simulink model "IK_PickPlaceTrajectory"  (R2023a)
settings: Solver=VariableStepAuto  StartTime=0.0  StopTime=10.0  RelTol=1e-3
values from neighbouring files (symbols this model uses):
  m = [4.043687892216430,4.088351020081470,2.975514330882000,2.005251413706830,1.580964077451070,0.312204788418883]    [Alternative_Approach_for_Jacobian.m]    (also in Dynamics6DOF_code.m)
undefined symbols (not defined in the file or in its folder): B, Spline, X, Y, Z
libraries: sm_lib x61, nesl_utility x19, robotcorelib x3, robotmaniplib x1
(part 2 of 2)

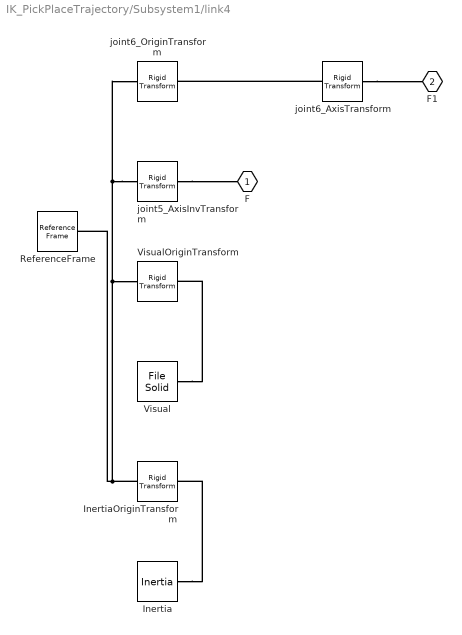
== system IK_PickPlaceTrajectory/Subsystem1/link4 ==
  Inertia : sm_lib/Body Elements/Inertia  InertiaType=Custom  Mass=1.93952788406336  MassUnits=kg  CenterOfMass=[0, 0, 0]  CenterOfMassUnits=m  MomentsOfInertia=[0.00155390886602976, 0.00197625240925502, 0.00139914012504898]  MomentsOfInertiaUnits=kg*m^2  ProductsOfInertia=[-0.000238629251977827, 2.66730188215764e-06, -2.69206560401887e-06]  ProductsOfInertiaUnits=kg*m^2  GraphicType=None  MarkerShape=Inertia  MarkerSize=20  GraphicVisPropType=SimpleVisualProperties  GraphicDiffuseColor=[0.5 0.5 0.5]  GraphicSpecularColor=[0.5 0.5 0.5 1.0]  GraphicAmbientColor=[0.15 0.15 0.15 1.0]  GraphicEmissiveColor=[0.0 0.0 0.0 1.0]  GraphicShininess=75  GraphicOpacity=1.0
  InertiaOriginTransform : sm_lib/Frames and Transforms/Rigid Transform  TranslationMethod=Cartesian  TranslationStandardOffset=0  TranslationStandardOffsetUnits=m  TranslationStandardAxis=+Z  TranslationCartesianOffset=[0.00193589454404341, 0.0412277276852661, -0.00711984165498196]  TranslationCartesianOffsetUnits=m  TranslationROffset=0  TranslationROffsetUnits=m  TranslationZOffset=0  TranslationZOffsetUnits=m  TranslationThetaOffset=0  TranslationThetaOffsetUnits=deg  RotationMethod=RotationSequence  RotationAngleUnits=deg  RotationStandardAxis=+Z  RotationAngle=0.0  RotationArbitraryAxis=[0 0 1]  FollAlignAxisA=+X  BaseAlignAxisA=+Y  FollAlignAxisB=+Y  BaseAlignAxisB=+Z  RotationSequenceAxes=BaseAxes  RotationSequence=XYZ  RotationSequenceAngles=[0, 0, 0]  RotationSequenceAnglesUnits=rad  RotationMatrix=[1 0 0; 0 1 0; 0 0 1]  Quaternion=[1 0 0 0]
  ReferenceFrame : sm_lib/Frames and Transforms/Reference Frame
  Visual : sm_lib/Body Elements/File Solid  ExtGeomFileName=PickandPlace_Assembly/meshes/link4.STL  UnitType=Custom  ExtGeomFileUnits=m  StepReaderType=HEX  ExportConvexHullGeometry=off  InertiaType=Custom  Mass=0  MassUnits=kg  CenterOfMass=[0, 0, 0]  CenterOfMassUnits=m  MomentsOfInertia=[0, 0, 0]  MomentsOfInertiaUnits=kg*m^2  ProductsOfInertia=[0, 0, 0]  ProductsOfInertiaUnits=kg*m^2  BasedOnType=DensityFromFile  Density=1000  DensityUnits=kg/m^3  DoExposeReferenceFrame=on  SerializedFrames=<Frames/>  GraphicType=FromGeometry  MarkerShape=Sphere  MarkerSize=10  GraphicVisPropType=SimpleVisualProperties  GraphicDiffuseColor=[0.752941176470588, 0.752941176470588, 0.752941176470588]  GraphicSpecularColor=[0.5 0.5 0.5 1.0]  GraphicAmbientColor=[0.15 0.15 0.15 1.0]  GraphicEmissiveColor=[0.0 0.0 0.0 1.0]  GraphicShininess=75  GraphicOpacity=1
  VisualOriginTransform : sm_lib/Frames and Transforms/Rigid Transform  TranslationMethod=Cartesian  TranslationStandardOffset=0  TranslationStandardOffsetUnits=m  TranslationStandardAxis=+Z  TranslationCartesianOffset=[0, 0, 0.132]  TranslationCartesianOffsetUnits=m  TranslationROffset=0  TranslationROffsetUnits=m  TranslationZOffset=0  TranslationZOffsetUnits=m  TranslationThetaOffset=0  TranslationThetaOffsetUnits=deg  RotationMethod=RotationSequence  RotationAngleUnits=deg  RotationStandardAxis=+Z  RotationAngle=0.0  RotationArbitraryAxis=[0 0 1]  FollAlignAxisA=+X  BaseAlignAxisA=+Y  FollAlignAxisB=+Y  BaseAlignAxisB=+Z  RotationSequenceAxes=BaseAxes  RotationSequence=XYZ  RotationSequenceAngles=[0, 0, 0]  RotationSequenceAnglesUnits=rad  RotationMatrix=[1 0 0; 0 1 0; 0 0 1]  Quaternion=[1 0 0 0]
  joint5_AxisInvTransform : sm_lib/Frames and Transforms/Rigid Transform  TranslationMethod=Cartesian  TranslationStandardOffset=0  TranslationStandardOffsetUnits=m  TranslationStandardAxis=+Z  TranslationCartesianOffset=[0, 0, 0]  TranslationCartesianOffsetUnits=m  TranslationROffset=0  TranslationROffsetUnits=m  TranslationZOffset=0  TranslationZOffsetUnits=m  TranslationThetaOffset=0  TranslationThetaOffsetUnits=deg  RotationMethod=ArbitraryAxis  RotationAngleUnits=rad  RotationStandardAxis=+Z  RotationAngle=0  RotationArbitraryAxis=[1, 0, 0]  FollAlignAxisA=+X  BaseAlignAxisA=+Y  FollAlignAxisB=+Y  BaseAlignAxisB=+Z  RotationSequenceAxes=FollowerAxes  RotationSequence=XYX  RotationSequenceAngles=[0 0 0]  RotationSequenceAnglesUnits=deg  RotationMatrix=[1 0 0; 0 1 0; 0 0 1]  Quaternion=[1 0 0 0]
  joint6_AxisTransform : sm_lib/Frames and Transforms/Rigid Transform  TranslationMethod=Cartesian  TranslationStandardOffset=0  TranslationStandardOffsetUnits=m  TranslationStandardAxis=+Z  TranslationCartesianOffset=[0, 0, 0]  TranslationCartesianOffsetUnits=m  TranslationROffset=0  TranslationROffsetUnits=m  TranslationZOffset=0  TranslationZOffsetUnits=m  TranslationThetaOffset=0  TranslationThetaOffsetUnits=deg  RotationMethod=ArbitraryAxis  RotationAngleUnits=rad  RotationStandardAxis=+Z  RotationAngle=0  RotationArbitraryAxis=[1, 0, 0]  FollAlignAxisA=+X  BaseAlignAxisA=+Y  FollAlignAxisB=+Y  BaseAlignAxisB=+Z  RotationSequenceAxes=FollowerAxes  RotationSequence=XYX  RotationSequenceAngles=[0 0 0]  RotationSequenceAnglesUnits=deg  RotationMatrix=[1 0 0; 0 1 0; 0 0 1]  Quaternion=[1 0 0 0]
  joint6_OriginTransform : sm_lib/Frames and Transforms/Rigid Transform  TranslationMethod=Cartesian  TranslationStandardOffset=0  TranslationStandardOffsetUnits=m  TranslationStandardAxis=+Z  TranslationCartesianOffset=[0, 0, 0.132]  TranslationCartesianOffsetUnits=m  TranslationROffset=0  TranslationROffsetUnits=m  TranslationZOffset=0  TranslationZOffsetUnits=m  TranslationThetaOffset=0  TranslationThetaOffsetUnits=deg  RotationMethod=RotationSequence  RotationAngleUnits=deg  RotationStandardAxis=+Z  RotationAngle=0.0  RotationArbitraryAxis=[0 0 1]  FollAlignAxisA=+X  BaseAlignAxisA=+Y  FollAlignAxisB=+Y  BaseAlignAxisB=+Z  RotationSequenceAxes=BaseAxes  RotationSequence=XYZ  RotationSequenceAngles=[-1.5707963267949, 0, 0]  RotationSequenceAnglesUnits=rad  RotationMatrix=[1 0 0; 0 1 0; 0 0 1]  Quaternion=[1 0 0 0]
  F : PMIOPort  Side=Left
  F1 : PMIOPort  Port=2  Side=Right
  connections:
  Inertia/RConn1 -- InertiaOriginTransform/RConn1
  joint5_AxisInvTransform/LConn1 -- joint6_OriginTransform/LConn1 -- InertiaOriginTransform/LConn1 -- ReferenceFrame/RConn1 -- VisualOriginTransform/LConn1
  Visual/RConn1 -- VisualOriginTransform/RConn1
  joint5_AxisInvTransform/RConn1 -- F/RConn1
  joint6_AxisTransform/RConn1 -- F1/RConn1
  joint6_AxisTransform/LConn1 -- joint6_OriginTransform/RConn1

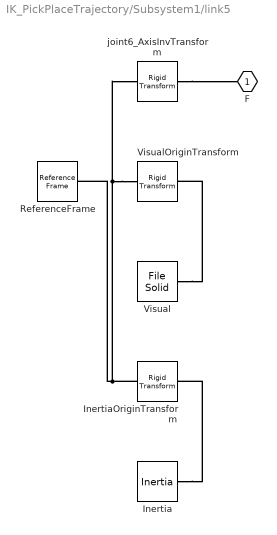
== system IK_PickPlaceTrajectory/Subsystem1/link5 ==
  Inertia : sm_lib/Body Elements/Inertia  InertiaType=Custom  Mass=0.312204788121022  MassUnits=kg  CenterOfMass=[0, 0, 0]  CenterOfMassUnits=m  MomentsOfInertia=[0.000111486628802788, 0.00017220756532504, 0.000149930296123144]  MomentsOfInertiaUnits=kg*m^2  ProductsOfInertia=[-2.62510399493773e-06, -6.16294543592803e-07, 1.09193037299933e-05]  ProductsOfInertiaUnits=kg*m^2  GraphicType=None  MarkerShape=Inertia  MarkerSize=20  GraphicVisPropType=SimpleVisualProperties  GraphicDiffuseColor=[0.5 0.5 0.5]  GraphicSpecularColor=[0.5 0.5 0.5 1.0]  GraphicAmbientColor=[0.15 0.15 0.15 1.0]  GraphicEmissiveColor=[0.0 0.0 0.0 1.0]  GraphicShininess=75  GraphicOpacity=1.0
  InertiaOriginTransform : sm_lib/Frames and Transforms/Rigid Transform  TranslationMethod=Cartesian  TranslationStandardOffset=0  TranslationStandardOffsetUnits=m  TranslationStandardAxis=+Z  TranslationCartesianOffset=[0.000634869948304639, 0.00391637711045545, 0.0604907685184927]  TranslationCartesianOffsetUnits=m  TranslationROffset=0  TranslationROffsetUnits=m  TranslationZOffset=0  TranslationZOffsetUnits=m  TranslationThetaOffset=0  TranslationThetaOffsetUnits=deg  RotationMethod=RotationSequence  RotationAngleUnits=deg  RotationStandardAxis=+Z  RotationAngle=0.0  RotationArbitraryAxis=[0 0 1]  FollAlignAxisA=+X  BaseAlignAxisA=+Y  FollAlignAxisB=+Y  BaseAlignAxisB=+Z  RotationSequenceAxes=BaseAxes  RotationSequence=XYZ  RotationSequenceAngles=[0, 0, 0]  RotationSequenceAnglesUnits=rad  RotationMatrix=[1 0 0; 0 1 0; 0 0 1]  Quaternion=[1 0 0 0]
  ReferenceFrame : sm_lib/Frames and Transforms/Reference Frame
  Visual : sm_lib/Body Elements/File Solid  ExtGeomFileName=PickandPlace_Assembly/meshes/link5.STL  UnitType=Custom  ExtGeomFileUnits=m  StepReaderType=HEX  ExportConvexHullGeometry=off  InertiaType=Custom  Mass=0  MassUnits=kg  CenterOfMass=[0, 0, 0]  CenterOfMassUnits=m  MomentsOfInertia=[0, 0, 0]  MomentsOfInertiaUnits=kg*m^2  ProductsOfInertia=[0, 0, 0]  ProductsOfInertiaUnits=kg*m^2  BasedOnType=DensityFromFile  Density=1000  DensityUnits=kg/m^3  DoExposeReferenceFrame=on  SerializedFrames=<Frames/>  GraphicType=FromGeometry  MarkerShape=Sphere  MarkerSize=10  GraphicVisPropType=SimpleVisualProperties  GraphicDiffuseColor=[0.752941176470588, 0.752941176470588, 0.752941176470588]  GraphicSpecularColor=[0.5 0.5 0.5 1.0]  GraphicAmbientColor=[0.15 0.15 0.15 1.0]  GraphicEmissiveColor=[0.0 0.0 0.0 1.0]  GraphicShininess=75  GraphicOpacity=1
  VisualOriginTransform : sm_lib/Frames and Transforms/Rigid Transform  TranslationMethod=Cartesian  TranslationStandardOffset=0  TranslationStandardOffsetUnits=m  TranslationStandardAxis=+Z  TranslationCartesianOffset=[0, 0, 0.050999]  TranslationCartesianOffsetUnits=m  TranslationROffset=0  TranslationROffsetUnits=m  TranslationZOffset=0  TranslationZOffsetUnits=m  TranslationThetaOffset=0  TranslationThetaOffsetUnits=deg  RotationMethod=RotationSequence  RotationAngleUnits=deg  RotationStandardAxis=+Z  RotationAngle=0.0  RotationArbitraryAxis=[0 0 1]  FollAlignAxisA=+X  BaseAlignAxisA=+Y  FollAlignAxisB=+Y  BaseAlignAxisB=+Z  RotationSequenceAxes=BaseAxes  RotationSequence=XYZ  RotationSequenceAngles=[0, 0, 0]  RotationSequenceAnglesUnits=rad  RotationMatrix=[1 0 0; 0 1 0; 0 0 1]  Quaternion=[1 0 0 0]
  joint6_AxisInvTransform : sm_lib/Frames and Transforms/Rigid Transform  TranslationMethod=Cartesian  TranslationStandardOffset=0  TranslationStandardOffsetUnits=m  TranslationStandardAxis=+Z  TranslationCartesianOffset=[0, 0, 0]  TranslationCartesianOffsetUnits=m  TranslationROffset=0  TranslationROffsetUnits=m  TranslationZOffset=0  TranslationZOffsetUnits=m  TranslationThetaOffset=0  TranslationThetaOffsetUnits=deg  RotationMethod=ArbitraryAxis  RotationAngleUnits=rad  RotationStandardAxis=+Z  RotationAngle=0  RotationArbitraryAxis=[1, 0, 0]  FollAlignAxisA=+X  BaseAlignAxisA=+Y  FollAlignAxisB=+Y  BaseAlignAxisB=+Z  RotationSequenceAxes=FollowerAxes  RotationSequence=XYX  RotationSequenceAngles=[0 0 0]  RotationSequenceAnglesUnits=deg  RotationMatrix=[1 0 0; 0 1 0; 0 0 1]  Quaternion=[1 0 0 0]
  F : PMIOPort  Side=Left
  connections:
  Inertia/RConn1 -- InertiaOriginTransform/RConn1
  VisualOriginTransform/LConn1 -- joint6_AxisInvTransform/LConn1 -- InertiaOriginTransform/LConn1 -- ReferenceFrame/RConn1
  Visual/RConn1 -- VisualOriginTransform/RConn1
  joint6_AxisInvTransform/RConn1 -- F/RConn1

== matlab function IK_PickPlaceTrajectory/MATLAB Function3 ==
  data: px input; th1_I_d output; py input; pz input; r11 input; th2_I_d output; th3_I_d output; th4_I_d output; th5_I_d output; th6_I_d output; r12 input; r13 input; r21 input; r22 input; r23 input; r31 input; r32 input; r33 input
function [th1_I_d, th2_I_d, th3_I_d, th4_I_d, th5_I_d, th6_I_d] = IF6(px, py, pz, r11, r12, r13, r21, r22, r23, r31, r32, r33)

    T_target = [r11 r12 r13 px; r21 r22 r23 py; r31 r32 r33 pz; 0 0 0 1];
    T_target = single(T_target);

    % DH parameters (lengths and offsets)
    d1 = 0.179; a2 = 0.410; a3 = 0.340; d4 = 0.188; d5 = 0.132; d6 = 0.00;
    
    % Joint Limits
    jointLimits = [
        -pi, pi;     % th1
         0, pi;   % th2
        -pi,0;     % th3
        -pi, pi;     % th4
        -pi, pi;     % th5
        -pi, pi;     % th6
    ];
    
    minError = single(inf);
    bestAngles = [0, 0, 0, 0, 0, 0];
    
    % Loop through each condition to calculate joint angles
    for condition = 1:8
        % Calculate th1 based on the current condition
        [th1, valid] = calcTheta1(px, py,d4,d6,r23,r13, condition);
        if ~valid, continue; end
        
        % Compute intermediate values for further calculations
        C = (cos(th1) * r11) + (sin(th1) * r21);
        D = (cos(th1) * r22) - (sin(th1) * r12);
        E = (sin(th1) * r11) - (cos(th1) * r21);
        
        % Calculate th5 based on the current condition
        [th5, valid] = calcTheta5(E, D, th1, r13, r23, condition);
        if ~valid, continue; end
        
        % Calculate th6 using trigonometric relationships
        th6 = atan2((D / sin(th5)), (E / sin(th5)));
        
        % Calculate th234 based on intermediate values
        F = cos(th5) * cos(th6);
        th234 = atan2(r31 * F - sin(th6) * C, F * C + sin(th6) * r31);
        
        Kc = cos(th1) * px + sin(th1) * py - sin(th234) * d5 + cos(th234) * sin(th5) * d6;
        Ks = pz - d1 + cos(th234) * d5 + sin(th234) * sin(th5) * d6;
        
        % Calculate th3 based on the current condition
        [th3] = calcTheta3(Ks, Kc, a2, a3, condition);
        
        % Calculate th2 and th4 based on intermediate values
        th2 = atan2(Ks, Kc) - atan2(sin(th3) * a3, cos(th3) * a3 + a2);
        th4 = th234 - th2 - th3;
        % For simplicity, let's assume a fixed time interval (dt)
        
        % Check joint constraints
        if ~checkJointConstraints([th1, th2, th3, th4, th5, th6], jointLimits)
            continue;
        end
        
        % Validate the solution using forward kinematics
        [T_calculated] = forward6DOF(th1, th2, th3, th4, th5, th6);
        
        % Compute the error between the calculated and target matrices
        error = norm(T_target - T_calculated, 'fro'); % Frobenius norm

        % Update the best solution if the current one is better
        if error < minError
            minError = error;
            bestAngles = [th1, th2, th3, th4, th5, th6]
            
        end
    end
    
    % Assign the best angles to the output variables
    th1_I_d = bestAngles(1);
    th2_I_d = bestAngles(2);
    th3_I_d = bestAngles(3);
    th4_I_d = bestAngles(4);
    th5_I_d = bestAngles(5);
    th6_I_d = bestAngles(6);

end

function [th1, valid] = calcTheta1(px, py, d4,d6,r23,r13, condition)
    A = py-d6*r23 ; % Adjusted for simplicity
    B = px-d6*r13; % Adjusted for simplicity
    root_th1 = B^2 + (-A)^2 - d4^2;
    valid = root_th1 >= 0;
    if valid
        th1_pos = atan2(sqrt(root_th1), d4) + atan2(B, -A);
        th1_neg = -atan2(sqrt(root_th1), d4) + atan2(B, -A);
        if condition == 1 || condition == 6 || condition == 7 || condition == 8
            th1 = th1_pos;
        else
            th1 = th1_neg;
        end
    else
        th1 = 0;
    end
end

function [th5, valid] = calcTheta5(E, D, th1, r13, r23, condition)
    root_th5 = E^2 + D^2;
    valid = root_th5 >= 0;
    if valid
        th5_pos = atan2(sqrt(root_th5), (sin(th1) * r13 - cos(th1) * r23));
        th5_neg = -atan2(sqrt(root_th5), (sin(th1) * r13 - cos(th1) * r23));
        if condition == 1 || condition == 2 || condition == 3 || condition == 6
            th5 = th5_pos;
        else
            th5 = th5_neg;
        end
    else
        th5 = 0;
    end
end

function [th3] = calcTheta3(Ks, Kc, a2, a3, condition)
    c3 = (Ks^2 + Kc^2 - a2^2 - a3^2) / (2 * a2 * a3);
    c3 = max(min(c3, 1), -1);
    s3 = sqrt(1 - c3^2);
    
    if condition == 1 || condition == 2 || condition == 4 || condition == 7
        th3 = atan2(s3, c3);
    else
        th3 = -atan2(s3, c3);
    end
end

% Function to check if the angles are within joint constraints
function valid = checkJointConstraints(angles, jointLimits)
    valid = true;
    for i = 1:length(angles)
        if angles(i) < jointLimits(i, 1) || angles(i) > jointLimits(i, 2)
            valid = false;
            break;
        end
    end
end
% Function to perform forward kinematics for a 6-DOF robot
function T2 = forward6DOF(th1, th2, th3, th4, th5, th6)
    d1 = 0.179; a2 = 0.410; a3 = 0.340; d4 = 0.188; d5 = 0.132; d6 = 0.00;
   
    c1 = cos(th1); c2 = cos(th2); c5 = cos(th5); c6 = cos(th6);
    s1 = sin(th1); s2 = sin(th2); s5 = sin(th5); s6 = sin(th6);
    c234 = cos(th2 + th3 + th4); s234 = sin(th2 + th3 + th4); c23 = cos(th2 + th3); s23 = sin(th2 + th3);
    r11 = (c1 * c234 * c5 * c6) + (c6 * s1 * s5) - (c1 * s234 * s6);
    r21 = (c234 * c5 * c6 * s1) - (c1 * c6 * s5) - (s1 * s234 * s6);
    r31 = (c5 * c6 * s234) + (c234 * s6);
    r12 = (-c1 * c234 * c5 * s6) - (s1 * s5 * s6) - (c1 * c6 * s234);
    r22 = (-c234 * c5 * s1 * s6) + (c1 * s5 * s6) - (c6 * s1 * s234);
    r32 = (-c5 * s234 * s6) + (c234 * c6);
    r13 = (-c1 * c234 * s5) + (c5 * s1);
    r23 = (-c234 * s1 * s5) - (c1 * c5);
    r33 = -s234 * s5;
    px = r13 * d6 + c1 * (s234 * d5 + c23 * a3 + c2 * a2) + s1 * d4;
    py = r23 * d6 + s1 * (s234 * d5 + c23 * a3 + c2 * a2) - c1 * d4;
    pz = r33 * d6 - c234 * d5 + s23 * a3 + s2 * a2 + d1;

    T2 = [r11 r12 r13 px; r21 r22 r23 py; r31 r32 r33 pz; 0 0 0 1];
end
